simulink model "DDSRF_PLL_test"  (R2025a)
settings: Solver=FixedStepAuto  StartTime=0.0  StopTime=0.2  FixedStep=sample_time_s_d  RelTol=1e-3  EnableMultiTasking=on
values from neighbouring files (symbols this model uses):
  filter_omega_out_a = single((2*pi*lpf_freq_out_cutoff_hz*sample_time_s))    [SRF_Config.m]
  filter_omega_out_b = single((1-(2*pi*lpf_freq_out_cutoff_hz*sample_time_s)))    [SRF_Config.m]
  filter_omega_out_init = single(filter_omega_out_a * grid_frequency_hz/(lpf_freq_out_cutoff_hz*sample_time_s))    [SRF_Config.m]
  filter_rms_out_a = single((2*pi*lpf_rms_out_cutoff_hz*sample_time_s))    [SRF_Config.m]
  filter_rms_out_b = single((1-(2*pi*lpf_rms_out_cutoff_hz*sample_time_s)))    [SRF_Config.m]
  filter_rms_out_init = single(220)    [SRF_Config.m]
  grid_frequency_hz = single(50)    [SRF_Config.m]
  pll_sat_max = single(150000)    [SRF_Config.m]
  pll_sat_min = single(-150000)    [SRF_Config.m]
  SRF_PI_I = single((2*pll_bandwidth_hz*pi)^2)    [SRF_Config.m]
  SRF_PI_P = single(2*2*pi*pll_bandwidth_hz*damping_factor_zeta)    [SRF_Config.m]
undefined symbols (not defined in the file or in its folder): DiscIntNeverNeededParam, dspblkCoreblockFVToolHelper, gcbh
libraries: simulink x2, mcbeeMathTransformLib x2, eeDiscretePi x1, spsabctoAlphaBetaZeroLib x1, spsdq0toabcLib x1
settings Model: Creator=Masood  LastModifiedBy=li_hh
settings OptimizationCC: DefaultParameterBehavior=Inlined  EnhancedBackFolding=on  PassReuseOutputArgsAs=Individual arguments  ZeroExternalMemoryAtStartup=off  MaxStackSize=2560  OptimizeBlockOrder=speed  DifferentSizesBufferReuse=on  OptimizationCustomize=off  EfficientTunableParamExpr=on
settings DebuggingCC: ParameterTunabilityLossMsg=error
settings HardwareCC: ProdBitPerPointer=32.0  ProdBitPerSizeT=32.0  ProdBitPerPtrDiffT=32.0  ProdLargestAtomicInteger=Long  ProdLargestAtomicFloat=Double  ProdWordSize=32.0  ProdHWDeviceType=ARM Compatible->ARM Cortex-M
settings SFSimCC: MATLABDynamicMemAlloc=off
settings RTWCC: SystemTargetFile=ert.tlc  TemplateMakefile=ert_default_tmf  Toolchain=Texas Instruments Code Composer Studio (ARM)  Description=Embedded Coder
settings CodeAppCC: ForceParamTrailComments=on  IgnoreCustomStorageClasses=off  OperatorAnnotations=on  SimulinkDataObjDesc=on  SFDataObjDesc=on  InsertBlockDesc=on
settings ERTTargetCC: ExtModeTransport=3.0  ERTCustomFileTemplate=example_file_process.tlc

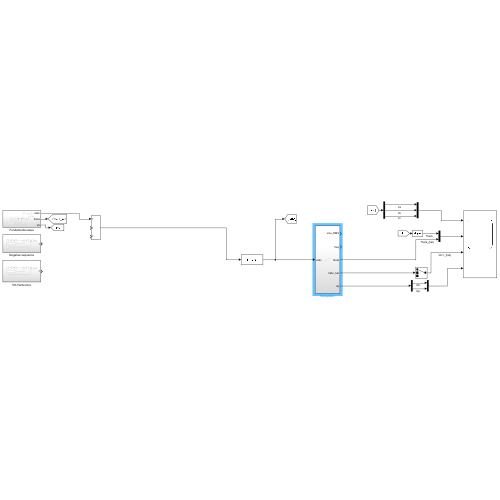
[thumbnail: Simulink's stored preview of the top-level diagram]
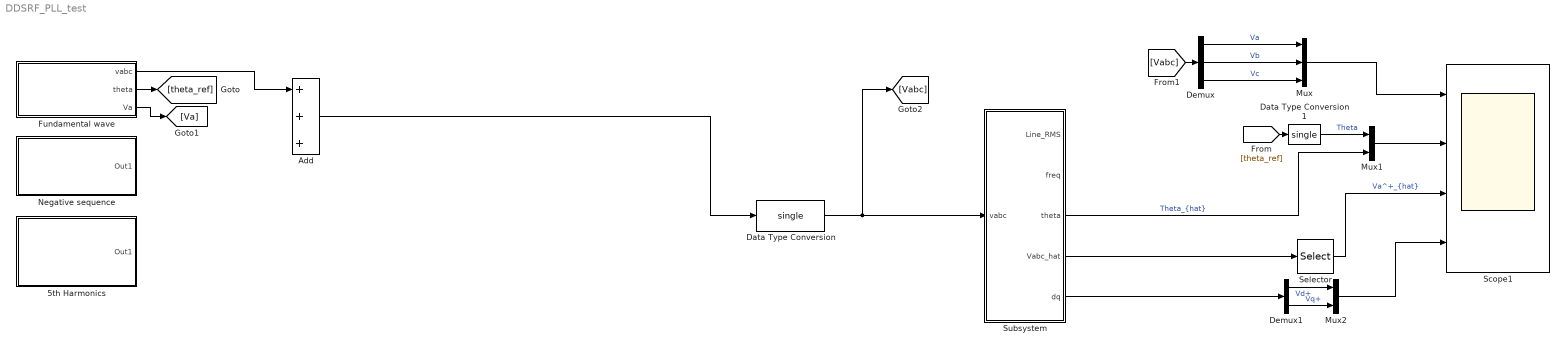
== system DDSRF_PLL_test ==
  5th Harmonics : Subsystem
  Add : Sum  Inputs=+++
  Data Type Conversion : DataTypeConversion  OutDataTypeStr=single  SaturateOnIntegerOverflow=off  RndMeth=Floor
  Data Type Conversion1 : DataTypeConversion  OutDataTypeStr=single  SaturateOnIntegerOverflow=off  RndMeth=Floor
  Demux : Demux  Outputs=3
  Demux1 : Demux  Outputs=2
  Fundamental wave : Subsystem
  Mux : Mux  Inputs=3
  Mux1 : Mux  Inputs=2
  Mux2 : Mux  Inputs=2
  Negative sequence : Subsystem
  Scope1 : Scope  NumInputPorts=4
      settings: ActiveDisplayYMinimum=-0.78539812564849831  ActiveDisplayYMaximum=7.0685831308364868  YLabel=Voltage/V
  Selector : Selector  InputPortWidth=3  IndexOptions=Index vector (dialog)  Indices=[1]  OutputSizes=1
  Subsystem : Subsystem
  wires:
  Fundamental wave/3(Va) -> [Va]
  Fundamental wave/2(theta) -> [theta_ref]
  Fundamental wave/1(vabc) -> Add/1
  Add/1 -> Data Type Conversion/1
  Data Type Conversion/1 -> [Vabc], Subsystem/1(vabc)
  Subsystem/4(Vabc_hat) -> Selector/1
  [Vabc] -> Demux/1
  Mux2/1 -> Scope1/4
  [theta_ref] -> Data Type Conversion1/1
  Demux1/2 -> Mux2/2  "Vq+"
  Mux1/1 -> Scope1/2
  Demux/1 -> Mux/1  "Va"
  Mux/1 -> Scope1/1
  Subsystem/3(theta) -> Mux1/2  "Theta_{hat}"
  Demux/2 -> Mux/2  "Vb"
  Subsystem/5(dq) -> Demux1/1
  Data Type Conversion1/1 -> Mux1/1  "Theta"
  Selector/1 -> Scope1/3  "Va^+_{hat}"
  Demux/3 -> Mux/3  "Vc"
  Demux1/1 -> Mux2/1  "Vd+"

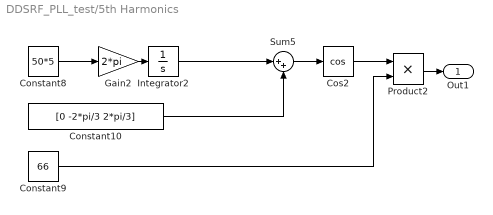
== system DDSRF_PLL_test/5th Harmonics ==
  Constant10 : Constant  Value=[0 -2*pi/3 2*pi/3]
  Constant8 : Constant  Value=50*5
  Constant9 : Constant  Value=66
  Cos2 : Trigonometry  Operator=cos
  Gain2 : Gain  Gain=2*pi
  Integrator2 : Integrator
  Product2 : Product
  Sum5 : Sum  Inputs=|++
  Out1 : Outport
  wires:
  Constant8/1 -> Gain2/1
  Constant9/1 -> Product2/2
  Cos2/1 -> Product2/1
  Product2/1 -> Out1/1
  Constant10/1 -> Sum5/2
  Integrator2/1 -> Sum5/1
  Gain2/1 -> Integrator2/1
  Sum5/1 -> Cos2/1

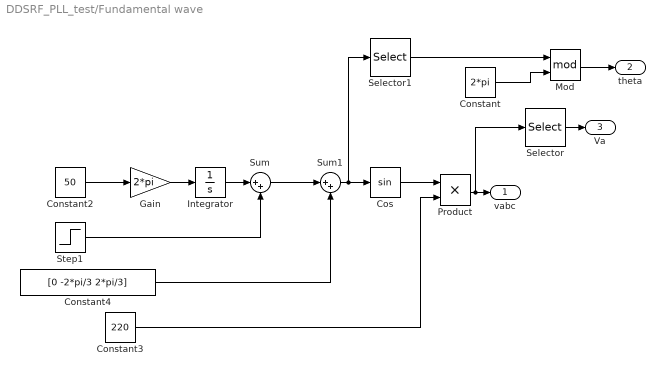
== system DDSRF_PLL_test/Fundamental wave ==
  Constant : Constant  Value=2*pi
  Constant2 : Constant  Value=50
  Constant3 : Constant  Value=220
  Constant4 : Constant  Value=[0 -2*pi/3 2*pi/3]
  Cos : Trigonometry
  Gain : Gain  Gain=2*pi
  Integrator : Integrator
  Mod : Math  Operator=mod
  Product : Product
  Selector : Selector  InputPortWidth=3  IndexOptions=Index vector (dialog)  Indices=[1]  OutputSizes=1
  Selector1 : Selector  InputPortWidth=3  IndexOptions=Index vector (dialog)  Indices=[1]  OutputSizes=1
  Step1 : Step  Time=0.1  After=-pi
  Sum : Sum  Inputs=|++
  Sum1 : Sum  Inputs=|++
  vabc : Outport
  theta : Outport  Port=2
  Va : Outport  Port=3
  wires:
  Step1/1 -> Sum/2
  Cos/1 -> Product/1
  Integrator/1 -> Sum/1
  Sum1/1 -> Selector1/1, Cos/1
  Constant3/1 -> Product/2
  Constant4/1 -> Sum1/2
  Sum/1 -> Sum1/1
  Constant2/1 -> Gain/1
  Product/1 -> Selector/1, vabc/1
  Gain/1 -> Integrator/1
  Selector/1 -> Va/1
  Mod/1 -> theta/1
  Constant/1 -> Mod/2
  Selector1/1 -> Mod/1

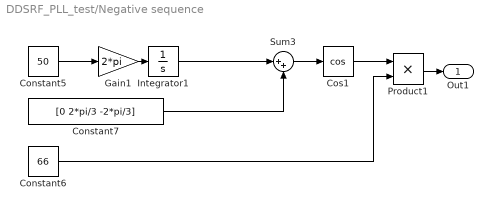
== system DDSRF_PLL_test/Negative sequence ==
  Constant5 : Constant  Value=50
  Constant6 : Constant  Value=66
  Constant7 : Constant  Value=[0 2*pi/3 -2*pi/3]
  Cos1 : Trigonometry  Operator=cos
  Gain1 : Gain  Gain=2*pi
  Integrator1 : Integrator
  Product1 : Product
  Sum3 : Sum  Inputs=|++
  Out1 : Outport
  wires:
  Integrator1/1 -> Sum3/1
  Cos1/1 -> Product1/1
  Constant7/1 -> Sum3/2
  Constant6/1 -> Product1/2
  Gain1/1 -> Integrator1/1
  Constant5/1 -> Gain1/1
  Product1/1 -> Out1/1
  Sum3/1 -> Cos1/1

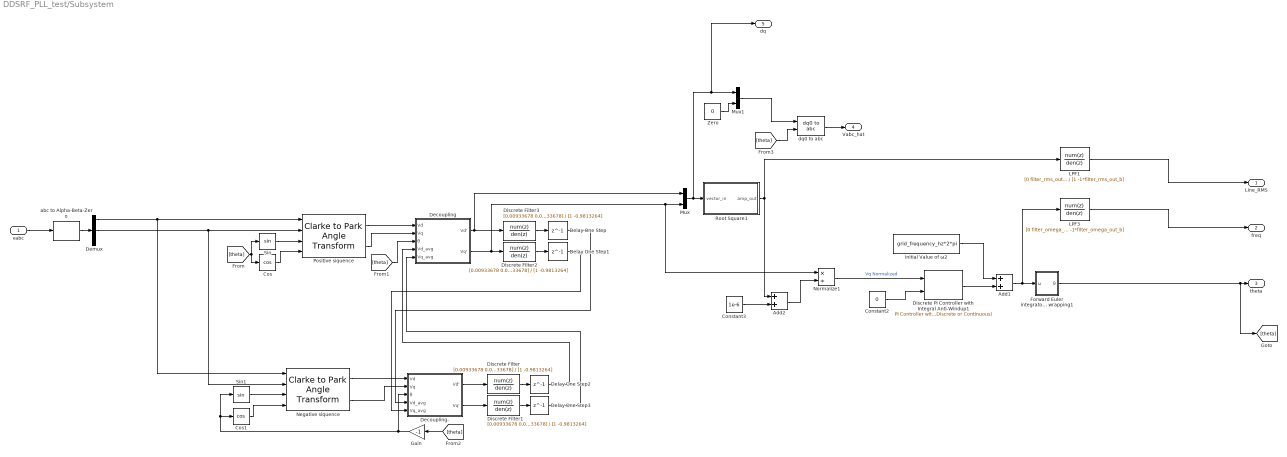
== system DDSRF_PLL_test/Subsystem ==
  vabc : Inport
  Add1 : Sum
  Add2 : Sum  OutDataTypeStr=single
  Constant2 : Constant  Value=0  OutDataTypeStr=single
  Constant3 : Constant  Value=1e-6  OutDataTypeStr=single
  Cos : Trigonometry  Operator=cos
  Cos1 : Trigonometry  Operator=cos
  Decoupling : Subsystem
  Decoupling- : Subsystem
  Delay One Step{,1..3} (4 alike) : Delay  DelayLength=1
  Demux : Demux  Outputs=3
  Discrete Filter{,1..3} (4 alike) : DiscreteFilter  LoadFcn=dspblkCoreblockFVToolHelper(gcbh,'load');  Numerator=[0.00933678 0.00933678]  Denominator=[1 -0.9813264]
      settings: CopyFcn=dspblkCoreblockFVToolHelper(gcbh,'copy');  DeleteFcn=dspblkCoreblockFVToolHelper(gcbh,'close');  ModelCloseFcn=dspblkCoreblockFVToolHelper(gcbh,'close');  PreSaveFcn=dspblkCoreblockFVToolHelper(gcbh,'presave');  PostSaveFcn=dspblkCoreblockFVToolHelper(gcbh,'postsave');  CloseFcn=dspblkCoreblockFVToolHelper(gcbh,'close');
  Discrete PI Controller with Integral Anti-Windup1 : eeDiscretePi/PI Controller with Integral Anti-Windup (Discrete or Continuous)  Kp=SRF_PI_P  Ki=SRF_PI_I  x0=0  B=pll_sat_max  A=pll_sat_min  Ts=-1
  Forward Euler integrator 2π wrapping1 : Subsystem
  Gain : Gain  Gain=-1
  LPF1 : DiscreteFilter  LoadFcn=dspblkCoreblockFVToolHelper(gcbh,'load');  Numerator=[0 filter_rms_out_a]  Denominator=[1 -1*filter_rms_out_b]  InitialStates=filter_rms_out_init/filter_rms_out_a
      settings: CopyFcn=dspblkCoreblockFVToolHelper(gcbh,'copy');  DeleteFcn=dspblkCoreblockFVToolHelper(gcbh,'close');  ModelCloseFcn=dspblkCoreblockFVToolHelper(gcbh,'close');  PreSaveFcn=dspblkCoreblockFVToolHelper(gcbh,'presave');  PostSaveFcn=dspblkCoreblockFVToolHelper(gcbh,'postsave');  CloseFcn=dspblkCoreblockFVToolHelper(gcbh,'close');
  LPF3 : DiscreteFilter  LoadFcn=dspblkCoreblockFVToolHelper(gcbh,'load');  Numerator=[0 filter_omega_out_a]  Denominator=[1 -1*filter_omega_out_b]  InitialStates=filter_omega_out_init/filter_omega_out_a
      settings: CopyFcn=dspblkCoreblockFVToolHelper(gcbh,'copy');  DeleteFcn=dspblkCoreblockFVToolHelper(gcbh,'close');  ModelCloseFcn=dspblkCoreblockFVToolHelper(gcbh,'close');  PreSaveFcn=dspblkCoreblockFVToolHelper(gcbh,'presave');  PostSaveFcn=dspblkCoreblockFVToolHelper(gcbh,'postsave');  CloseFcn=dspblkCoreblockFVToolHelper(gcbh,'close');
  Mux : Mux  Inputs=2
  Mux1 : Mux  Inputs=2
  Negative siquence : mcbeeMathTransformLib/Clarke to Park Angle Transform  AxisAlignment=Q-axis  UseWithEmbedded=on  PhaseInput=Two inputs  ThetaInput=Sine and Cosine electrical position  AngleInput=Per-unit  N_points=1024
      settings: LibrarySourceBlock=mcbcontrolslib/Park Transform
  Normalize1 : Product  Inputs=*/
  Positive siquence : mcbeeMathTransformLib/Clarke to Park Angle Transform  AxisAlignment=Q-axis  UseWithEmbedded=on  PhaseInput=Two inputs  ThetaInput=Sine and Cosine electrical position  AngleInput=Per-unit  N_points=1024
      settings: LibrarySourceBlock=mcbcontrolslib/Park Transform
  Root Square1 : Subsystem
  Sin : Trigonometry
  Sin1 : Trigonometry
  Zero : Constant  Value=0  OutDataTypeStr=Inherit: Inherit via back propagation
  abc to Alpha-Beta-Zero : spsabctoAlphaBetaZeroLib/abc to Alpha-Beta-Zero
  dq0 to abc : spsdq0toabcLib/dq0 to abc  Alignment=90 degrees behind phase A axis
  initial Value of ω2 : Constant  Value=grid_frequency_hz*2*pi  OutDataTypeStr=single
  Line_RMS : Outport  OutDataTypeStr=single  PortDimensions=1
  freq : Outport  Port=2  OutDataTypeStr=single  PortDimensions=1
  theta : Outport  Port=3  OutDataTypeStr=single  PortDimensions=1
  Vabc_hat : Outport  Port=4
  dq : Outport  Port=5
  wires:
  Discrete PI Controller with Integral Anti-Windup1/1 -> Add1/2
  LPF3/1 -> freq/1
  initial Value of ω2/1 -> Add1/1
  Root Square1/1(amp_out) -> Add2/1, LPF1/1
  Normalize1/1 -> Discrete PI Controller with Integral Anti-Windup1/1  "Vq Normalized"
  Add1/1 -> LPF3/1, Forward Euler integrator 2π wrapping1/1(ω)
  Constant2/1 -> Discrete PI Controller with Integral Anti-Windup1/2
  Sin/1 -> Positive siquence/3
  Cos/1 -> Positive siquence/4
  Add2/1 -> Normalize1/2
  Constant3/1 -> Add2/2
  Demux/2 -> Negative siquence/2, Positive siquence/2
  LPF1/1 -> Line_RMS/1
  Forward Euler integrator 2π wrapping1/1(θ) -> [theta], theta/1
  Sin1/1 -> Negative siquence/3
  Cos1/1 -> Negative siquence/4
  Gain/1 -> Decoupling-/3(θ), Sin1/1, Cos1/1
  Positive siquence/1 -> Decoupling/1(Vd)
  Positive siquence/2 -> Decoupling/2(Vq)
  Negative siquence/1 -> Decoupling-/1(Vd)
  Negative siquence/2 -> Decoupling-/2(Vq)
  Decoupling/1(Vd') -> Mux/1, Discrete Filter3/1
  Decoupling/2(Vq') -> Normalize1/1, Mux/2, Discrete Filter2/1
  Decoupling-/1(Vd') -> Discrete Filter/1
  Decoupling-/2(Vq') -> Discrete Filter1/1
  Discrete Filter/1 -> Delay One Step2/1
  Discrete Filter1/1 -> Delay One Step3/1
  Discrete Filter3/1 -> Delay One Step/1
  Discrete Filter2/1 -> Delay One Step1/1
  Delay One Step/1 -> Decoupling-/4(Vd_avg)
  Delay One Step1/1 -> Decoupling-/5(Vq_avg)
  Delay One Step2/1 -> Decoupling/4(Vd_avg)
  Delay One Step3/1 -> Decoupling/5(Vq_avg)
  [theta] -> Sin/1, Cos/1
  [theta] -> Decoupling/3(θ)
  [theta] -> Gain/1
  Mux/1 -> dq/1, Mux1/1, Root Square1/1(vector_in)
  vabc/1 -> abc to Alpha-Beta-Zero/1
  abc to Alpha-Beta-Zero/1 -> Demux/1
  Demux/1 -> Negative siquence/1, Positive siquence/1
  [theta] -> dq0 to abc/2
  Zero/1 -> Mux1/2
  Mux1/1 -> dq0 to abc/1
  dq0 to abc/1 -> Vabc_hat/1

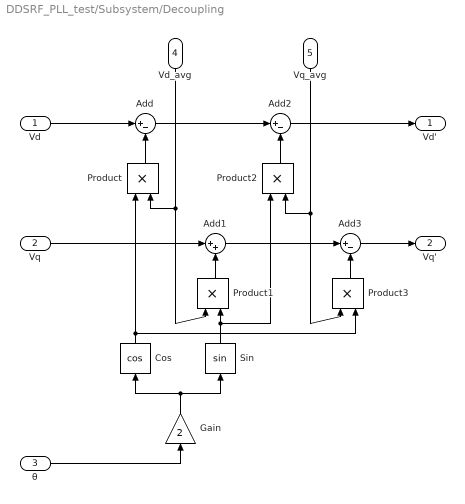
== system DDSRF_PLL_test/Subsystem/Decoupling ==
  Vd : Inport
  Vq : Inport  Port=2
  θ : Inport  Port=3
  Vd_avg : Inport  Port=4
  Vq_avg : Inport  Port=5
  Add : Sum  Inputs=|+-
  Add1 : Sum  Inputs=|++
  Add2 : Sum  Inputs=|+-
  Add3 : Sum  Inputs=|+-
  Cos : Trigonometry  Operator=cos
  Gain : Gain  Gain=2
  Product{,1..3} (4 alike) : Product
  Sin : Trigonometry
  Vd' : Outport
  Vq' : Outport  Port=2
  wires:
  θ/1 -> Gain/1
  Gain/1 -> Sin/1, Cos/1
  Cos/1 -> Product3/2, Product/1
  Product/1 -> Add/2
  Vd/1 -> Add/1
  Sin/1 -> Product2/1, Product1/2
  Vd_avg/1 -> Product/2, Product1/1
  Product1/1 -> Add1/2
  Vq/1 -> Add1/1
  Vq_avg/1 -> Product2/2, Product3/1
  Product2/1 -> Add2/2
  Add/1 -> Add2/1
  Add2/1 -> Vd'/1
  Product3/1 -> Add3/2
  Add1/1 -> Add3/1
  Add3/1 -> Vq'/1

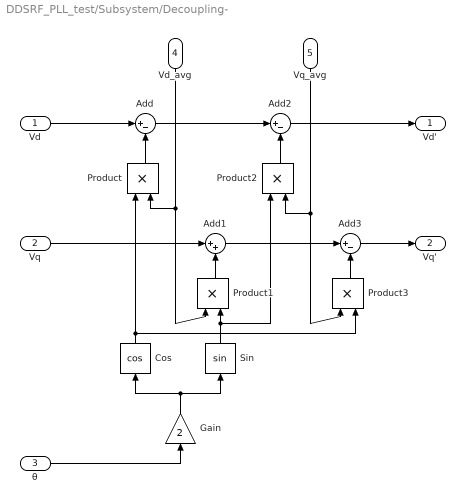
== system DDSRF_PLL_test/Subsystem/Decoupling- ==
  Vd : Inport
  Vq : Inport  Port=2
  θ : Inport  Port=3
  Vd_avg : Inport  Port=4
  Vq_avg : Inport  Port=5
  Add : Sum  Inputs=|+-
  Add1 : Sum  Inputs=|++
  Add2 : Sum  Inputs=|+-
  Add3 : Sum  Inputs=|+-
  Cos : Trigonometry  Operator=cos
  Gain : Gain  Gain=2
  Product{,1..3} (4 alike) : Product
  Sin : Trigonometry
  Vd' : Outport
  Vq' : Outport  Port=2
  wires:
  θ/1 -> Gain/1
  Gain/1 -> Sin/1, Cos/1
  Cos/1 -> Product3/2, Product/1
  Product/1 -> Add/2
  Vd/1 -> Add/1
  Sin/1 -> Product2/1, Product1/2
  Vd_avg/1 -> Product/2, Product1/1
  Product1/1 -> Add1/2
  Vq/1 -> Add1/1
  Vq_avg/1 -> Product2/2, Product3/1
  Product2/1 -> Add2/2
  Add/1 -> Add2/1
  Add2/1 -> Vd'/1
  Product3/1 -> Add3/2
  Add1/1 -> Add3/1
  Add3/1 -> Vq'/1

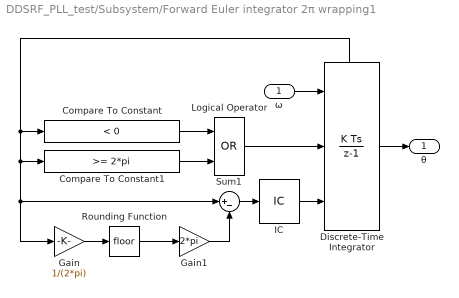
== system DDSRF_PLL_test/Subsystem/Forward Euler integrator 2π wrapping1 ==
  ω : Inport
  Compare To Constant : simulink/Logic and Bit Operations/Compare To Constant  relop=<  const=0  OutDataTypeStr=boolean
  Compare To Constant1 : simulink/Logic and Bit Operations/Compare To Constant  relop=>=  const=2*pi  OutDataTypeStr=boolean
  Discrete-Time Integrator : DiscreteIntegrator  ExternalReset=sampled level  InitialConditionSource=external  SampleTime=-1  OutDataTypeStr=single  ShowStatePort=on  ICPrevOutput=DiscIntNeverNeededParam  ICPrevScaledInput=DiscIntNeverNeededParam
  Gain : Gain  Gain=1/(2*pi)
      settings: AttributesFormatString=%<Gain>
  Gain1 : Gain  Gain=2*pi
  IC : InitialCondition  Value=0
  Logical Operator : Logic  Operator=OR  AllPortsSameDT=off  OutDataTypeStr=boolean
  Rounding Function : Rounding
  Sum1 : Sum  Inputs=|+-
  θ : Outport
  wires:
  Gain1/1 -> Sum1/2
  Gain/1 -> Rounding Function/1
  IC/1 -> Discrete-Time Integrator/3
  Compare To Constant1/1 -> Logical Operator/2
  Discrete-Time Integrator/State -> Compare To Constant1/1, Sum1/1, Gain/1, Compare To Constant/1
  Compare To Constant/1 -> Logical Operator/1
  Logical Operator/1 -> Discrete-Time Integrator/2
  Sum1/1 -> IC/1
  Rounding Function/1 -> Gain1/1
  ω/1 -> Discrete-Time Integrator/1
  Discrete-Time Integrator/1 -> θ/1

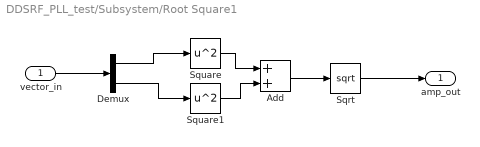
== system DDSRF_PLL_test/Subsystem/Root Square1 ==
  vector_in : Inport
  Add : Sum
  Demux : Demux  Outputs=2
  Sqrt : Sqrt
  Square : Math  Operator=square
  Square1 : Math  Operator=square
  amp_out : Outport
  wires:
  Square/1 -> Add/1
  Add/1 -> Sqrt/1
  Sqrt/1 -> amp_out/1
  Demux/2 -> Square1/1
  Square1/1 -> Add/2
  vector_in/1 -> Demux/1
  Demux/1 -> Square/1
